simulink model "single_area_model_P_control"  (R2014b)
settings: Solver=ode45  StartTime=0.0  StopTime=11.0  RelTol=1e-3
settings Model: Creator=Shane Reynolds  LastModifiedBy=Shane Reynolds

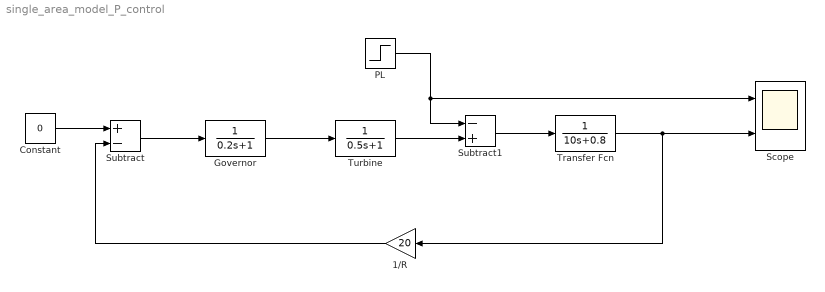
== system single_area_model_P_control ==
  1/R : Gain  Gain=20
  Constant : Constant  Value=0
  Governor : TransferFcn  Denominator=[0.2 1]
  PL : Step  After=0.2  SampleTime=0
  Scope : Scope  NumInputPorts=2
      settings: YMin=-1~-1  YMax=1~1
  Subtract : Sum  Inputs=+-
  Subtract1 : Sum  Inputs=-+
  Transfer Fcn : TransferFcn  Denominator=[10 0.8]
  Turbine : TransferFcn  Denominator=[0.5 1]
  wires:
  Governor/1 -> Turbine/1
  Subtract/1 -> Governor/1
  1/R/1 -> Subtract/2
  Turbine/1 -> Subtract1/2
  Subtract1/1 -> Transfer Fcn/1
  PL/1 -> Scope/1, Subtract1/1
  Transfer Fcn/1 -> Scope/2, 1/R/1
  Constant/1 -> Subtract/1
